simulink model "test_seance32"  (R2013b)
settings: Solver=ode4  StartTime=0.0  StopTime=0.0149  FixedStep=Te  RelTol=1e-3
undefined symbols (not defined in the file): Ka, Kb, Te
settings Model: Creator=gemsdev  LastModifiedBy=gemsdev

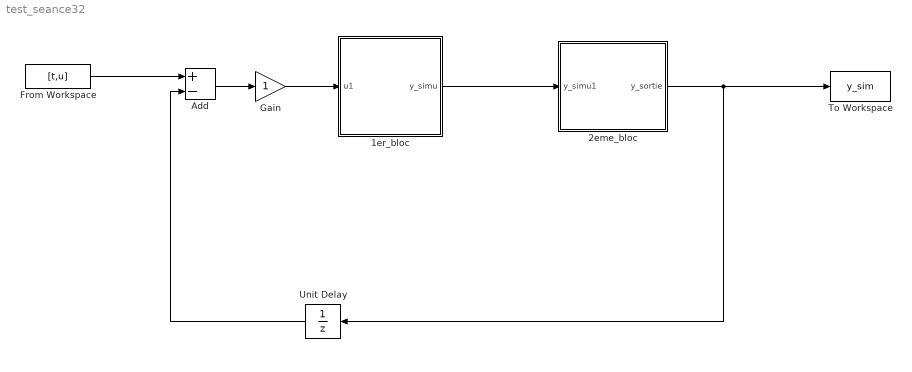
== system test_seance32 ==
  1er_bloc : Subsystem
  2eme_bloc : Subsystem
  Add : Sum  Inputs=+-
  From Workspace : FromWorkspace  VariableName=[t,u]  SampleTime=0
  Gain : Gain
  To Workspace : ToWorkspace  VariableName=y_sim  SampleTime=-1
  Unit Delay : UnitDelay  SampleTime=-1
  wires:
  2eme_bloc/1(y_sortie) -> To Workspace/1, Unit Delay/1
  1er_bloc/1(y_simu) -> 2eme_bloc/1(y_simu1)
  From Workspace/1 -> Add/1
  Add/1 -> Gain/1
  Unit Delay/1 -> Add/2
  Gain/1 -> 1er_bloc/1(u1)

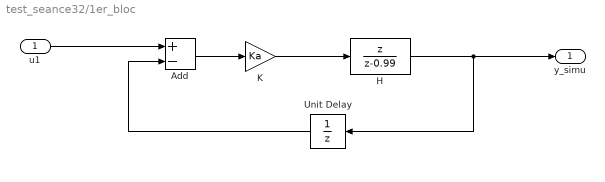
== system test_seance32/1er_bloc ==
  u1 : Inport
  Add : Sum  Inputs=+-  SampleTime=Te
  H : DiscreteTransferFcn  Numerator=[1 0]  Denominator=[1 -0.99]  SampleTime=Te
  K : Gain  Gain=Ka  SampleTime=Te
  Unit Delay : UnitDelay  SampleTime=Te
  y_simu : Outport
  wires:
  Add/1 -> K/1
  K/1 -> H/1
  H/1 -> y_simu/1, Unit Delay/1
  Unit Delay/1 -> Add/2
  u1/1 -> Add/1

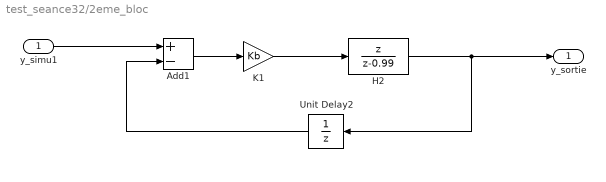
== system test_seance32/2eme_bloc ==
  y_simu1 : Inport
  Add1 : Sum  Inputs=+-  SampleTime=Te
  H2 : DiscreteTransferFcn  Numerator=[1 0]  Denominator=[1 -0.99]  SampleTime=Te
  K1 : Gain  Gain=Kb  SampleTime=Te
  Unit Delay2 : UnitDelay  SampleTime=Te
  y_sortie : Outport
  wires:
  y_simu1/1 -> Add1/1
  H2/1 -> y_sortie/1, Unit Delay2/1
  Add1/1 -> K1/1
  Unit Delay2/1 -> Add1/2
  K1/1 -> H2/1
